simulink model "lab2_1"  (R2022a)
settings: Solver=VariableStepAuto  StartTime=0.0  StopTime=20.0  RelTol=1e-3
settings Model: Creator=hyhung3  LastModifiedBy=hyhung3

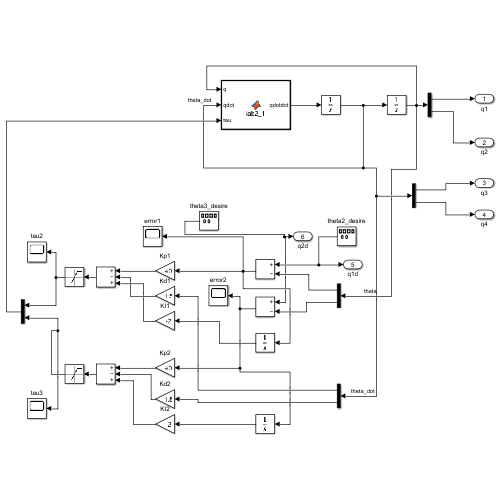
[thumbnail: Simulink's stored preview of the top-level diagram]
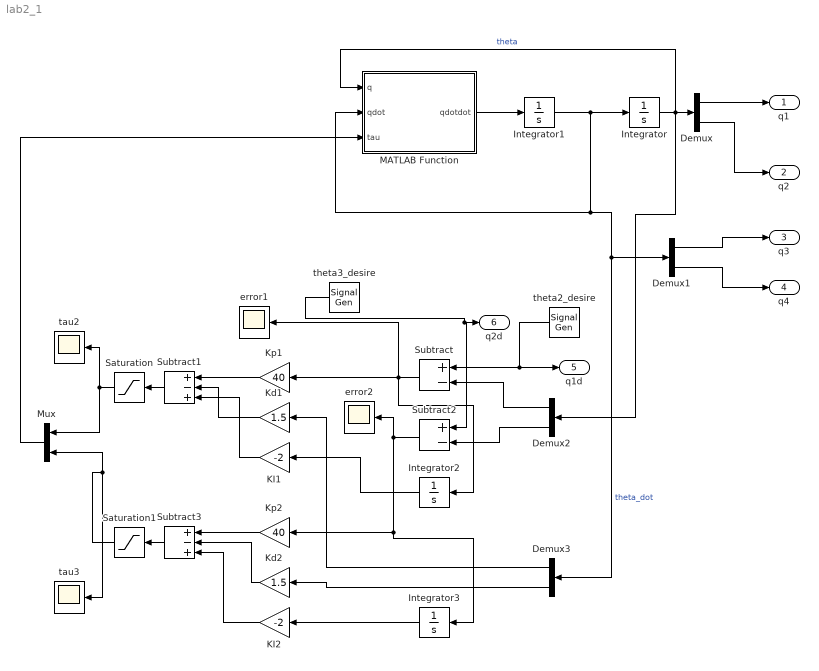
== system lab2_1 ==
  Demux{,1..3} (4 alike) : Demux  Outputs=2
  Integrator : Integrator  InitialCondition=[0;0]
  Integrator1 : Integrator  InitialCondition=[0;0]
  Integrator2 : Integrator
  Integrator3 : Integrator
  KI1 : Gain  Gain=-2
  KI2 : Gain  Gain=-2
  Kd1 : Gain  Gain=1.5
  Kd2 : Gain  Gain=1.5
  Kp1 : Gain  Gain=40
  Kp2 : Gain  Gain=40
  MATLAB Function : MATLAB Function  TreatAsAtomicUnit=on
  Mux : Mux  Inputs=2
  Saturation : Saturate  UpperLimit=5  LowerLimit=-5
  Saturation1 : Saturate  UpperLimit=5  LowerLimit=-5
  Subtract : Sum  Inputs=+-
  Subtract1 : Sum  Inputs=+-+
  Subtract2 : Sum  Inputs=+-
  Subtract3 : Sum  Inputs=+-+
  error1 : Scope
  error2 : Scope
  tau2 : Scope
  tau3 : Scope
  theta2_desire : SignalGenerator  WaveForm=square  Amplitude=0.25  Frequency=0.25
  theta3_desire : SignalGenerator  WaveForm=square  Amplitude=0.25  Frequency=0.25
  q1 : Outport
  q2 : Outport  Port=2
  q3 : Outport  Port=3
  q4 : Outport  Port=4
  q1d : Outport  Port=5
  q2d : Outport  Port=6
  wires:
  Integrator1/1 -> Integrator/1, Demux3/1, Demux1/1, MATLAB Function/2(qdot)  "theta_dot"
  Integrator/1 -> Demux2/1, MATLAB Function/1(q), Demux/1  "theta"
  MATLAB Function/1(qdotdot) -> Integrator1/1
  theta2_desire/1 -> Subtract/1, q1d/1
  Demux2/1 -> Subtract/2
  Subtract/1 -> Integrator2/1, Kp1/1, error1/1
  Demux3/1 -> Kd1/1
  Kd1/1 -> Subtract1/2
  Kp1/1 -> Subtract1/1
  Demux2/2 -> Subtract2/2
  Demux3/2 -> Kd2/1
  Kd2/1 -> Subtract3/2
  Kp2/1 -> Subtract3/1
  Mux/1 -> MATLAB Function/3(tau)
  theta3_desire/1 -> Subtract2/1, q2d/1
  Subtract1/1 -> Saturation/1
  Saturation/1 -> Mux/1, tau2/1
  Subtract3/1 -> Saturation1/1
  Saturation1/1 -> tau3/1, Mux/2
  Demux/2 -> q2/1
  Demux/1 -> q1/1
  Demux1/1 -> q3/1
  Demux1/2 -> q4/1
  Integrator2/1 -> KI1/1
  Subtract2/1 -> Integrator3/1, Kp2/1, error2/1
  Integrator3/1 -> KI2/1
  KI1/1 -> Subtract1/3
  KI2/1 -> Subtract3/3

== matlab function lab2_1/MATLAB Function ==
  data: q input; qdotdot output; qdot input; tau input
function qdotdot = lab2_1(q,qdot,tau)
g = 9.81;

theta2 = q(1);
theta3 = q(2);

theta2_dot = qdot(1);
theta3_dot = qdot(2);

p = [0.03; 0.0128; 0.0076; 0.0753; 0.0298];

p1 = p(1);
p2 = p(2);
p3 = p(3);
p4 = p(4);
p5 = p(5);

M = [[p1                        -p3*sin(theta3 - theta2)];
     [-p3*sin(theta3 - theta2)                        p2]];
C = [[0                                 -p3*cos(theta3 - theta2)*theta3_dot];
     [p3*cos(theta3 - theta2)*theta2_dot                                  0]];

G = [-p4*g*sin(theta2);
       -p5*g*cos(theta3)];

qdotdot = (inv(M))*tau - (inv(M))*C*qdot - (inv(M))*G;
